simulink model "Drone_helical_trajectory"  (R2024b)
settings: Solver=ode45  StartTime=0.0  StopTime=100  RelTol=1e-9  EnableMultiTasking=on
StopFcn:
  | x = X;
  | plot3(x(:,8), x(:,10), x(:,11), 'r-', LineWidth=1.5);
  | grid on;
settings Model: Creator=Dalil  LastModifiedBy=user
settings SolverCC: ZeroCrossAlgorithm=Adaptive  AlgebraicLoopSolver=TrustRegion
settings DataIOCC: LimitDataPoints=on  SaveFormat=Array  ReturnWorkspaceOutputs=off
settings OptimizationCC: ExpressionDepthLimit=2147483647  LifeSpan=inf
settings DebuggingCC: UnderspecifiedInitializationDetection=Classic  MergeDetectMultiDrivingBlocksExec=none  SolverPrmCheckMsg=warning  UnconnectedInputMsg=warning  UnconnectedOutputMsg=warning  UnconnectedLineMsg=warning  StateNameClashWarn=warning  SFUnexpectedBacktrackingDiag=warning  SFNoUnconditionalDefaultTransitionDiag=warning  SFExecutionAtInitializationDiag=none  ArithmeticOperatorsInVariantConditions=warning
settings HardwareCC: ProdBitPerPointer=32  ProdBitPerSizeT=32  ProdBitPerPtrDiffT=32  ProdLargestAtomicFloat=None  ProdIntDivRoundTo=Undefined  ProdEndianess=Unspecified  ProdWordSize=32  ProdHWDeviceType=32-bit Generic
settings ModelReferenceCC: EnableRefExpFcnMdlSchedulingChecks=on  PropagateSignalLabelsOutOfModel=off
settings SFSimCC: SimUseLocalCustomCode=off  CustomCodeUndefinedFunction=UseInterfaceOnly
settings RTWCC: RTWUseLocalCustomCode=off  GPUComputeCapability=3.5  DLArmComputeVersion=19.05
settings CodeAppCC: StateflowObjectComments=on
settings GRTTargetCC: TargetLangStandard=C89/C90 (ANSI)
settings ConfigComp: CovMetricSettings=dw  CovSaveCumulativeToWorkspaceVar=on  CovSaveSingleToWorkspaceVar=on  CovExternalEMLEnable=off

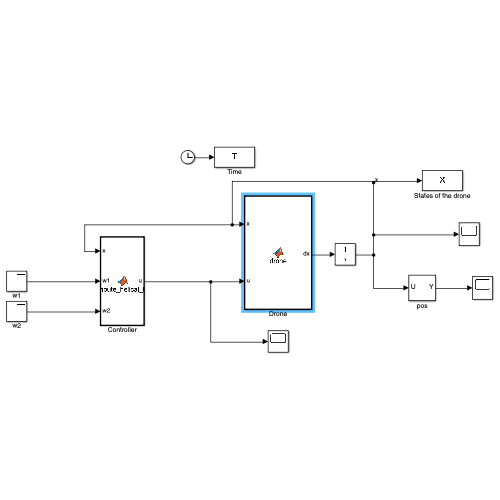
[thumbnail: Simulink's stored preview of the top-level diagram]
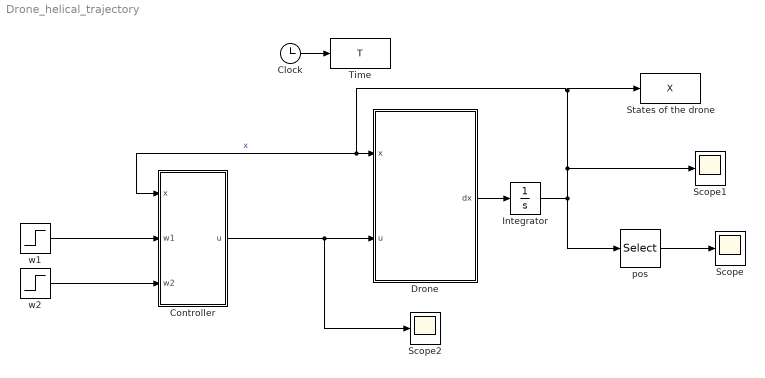
== system Drone_helical_trajectory ==
  Clock : Clock
  Controller : MATLAB Function  TreatAsAtomicUnit=on
  Drone : MATLAB Function  TreatAsAtomicUnit=on
  Integrator : Integrator  InitialCondition="[pi/6  0 pi/6 0 0 0 5 0  5 0 0 0]"  UpperSaturationLimit=[0 0 0 0 0 0 pi 0 pi 0 0 0]
  Scope : Scope
  Scope1 : Scope
  Scope2 : Scope
  States of the drone : ToWorkspace  VariableName=X  SampleTime=-1
  Time : ToWorkspace  VariableName=T  SampleTime=-1
  pos : Selector  InputPortWidth=12  IndexOptions=Index vector (dialog)  Indices=[5 8 10 11]  OutputSizes=1
  w1 : Step  Time=0  SampleTime=0
  w2 : Step  Time=0  After=2  SampleTime=0
  wires:
  Integrator/1 -> pos/1, Controller/1(x), Drone/1(x), States of the drone/1, Scope1/1  "x"
  Controller/1(u) -> Scope2/1, Drone/2(u)
  Clock/1 -> Time/1
  pos/1 -> Scope/1
  Drone/1(dx) -> Integrator/1
  w1/1 -> Controller/2(w1)
  w2/1 -> Controller/3(w2)

== matlab function Drone_helical_trajectory/Controller ==
  data: x input; w1 input; u output; w2 input
function u = compute_helical_trim(x, w1, w2)

    u = zeros(5,1);
    m=0.1; g=-9.81; b=1; d = 1;
    
    % control inputs for the model at helix conditions
    u(5) = 2*(w2 - w1);
    u(4) = m*g/(cos(x(1))*cos(x(3))) + m*x(12);
    u(3) = 2*d*(w2^2 - w1^2);
    u(2) = 0;
    u(1) = 0;
   
    
end

== matlab function Drone_helical_trajectory/Drone ==
  data: x input; u input; dx output
function dx = drone(x, u)
    % Parameters
    g = -9.81;         
    m = 0.10;          
    l = 0.25;         
    Ixx = 0.001;       
    Iyy = 0.001;       
    Izz = 0.002;       
    Jr = 0.01;        % Rotor inertia

    % Coefficients from the image
    a1 = (Iyy - Izz) / Ixx;
    a2 = Jr / Ixx;
    a3 = (Izz - Ixx) / Iyy;
    a4 = Jr / Iyy;
    a5 = (Ixx - Iyy) / Izz;

    b1 = l / Ixx;
    b2 = l / Iyy;
    b3 = l / Izz;

    % State variables
    % x(1) = phi, x(2) = phi_dot, x(3) = theta, x(4) = theta_dot,
    % x(5) = psi, x(6) = psi_dot, x(7) = x, x(8) = x_dot,
    % x(9) = y, x(10) = y_dot, x(11) = z, x(12) = z_dot

    % Control inputs
    U1 = u(1); % Roll moment
    U2 = u(2); % Pitch moment
    U3 = u(3); % Yaw moment
    U4 = u(4); % Collective thrust
    Ur = u(5); % Omega_r


    % State derivatives and conditions
    dx = zeros(12,1);
    %x(1)=0; x(3)=0;
    x(4)=x(2)== 0; %x(8)=x(10)==0;
    x(6) = pi/5; x(12) = 1;

    % Angular dynamics
    dx(1) = x(2);
    dx(2) = a1 * x(4) * x(6) + a2 * x(4) * Ur + b1 * U1; 
    dx(3) = x(4); 
    dx(4) = a3 * x(2) * x(6) - a4 * x(2) * Ur + b2 * U2; 
    dx(5) = pi/6; 
    dx(6) = 0; 

    % Translational dynamics
    dx(7) = x(8); 
    dx(8) = (U4 / m) * (cos(x(1)) * sin(x(3)) * cos(x(5)) + sin(x(1)) * sin(x(5))); 
    dx(9) = x(10); 
    dx(10) = (U4 / m) * (cos(x(1)) * sin(x(3)) * sin(x(5)) - sin(x(1)) * cos(x(5))); 
    dx(11) = x(12); 
    dx(12) = -g + (U4 / m) * (cos(x(1)) * cos(x(3)));

end
